simulink model "Paper_2_Model_2_fixed_delay_3_lines"  (R2020b)
settings: Solver=VariableStepAuto  StartTime=0.0  StopTime=3  RelTol=1e-3
libraries: simulink x1
settings Model: Creator=Isabel  LastModifiedBy=Isabel

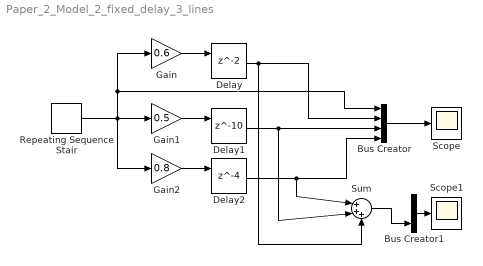
== system Paper_2_Model_2_fixed_delay_3_lines ==
  Bus Creator : BusCreator  Inputs=4
  Bus Creator1 : BusCreator  Inputs=2
  Delay : Delay  InitialConditionSource=Input port  InitialCondition=0  SampleTime=0.01
      settings: InputPortMap=u0,p4
  Delay1 : Delay  DelayLength=10  InitialConditionSource=Input port  InitialCondition=0  SampleTime=0.01
      settings: InputPortMap=u0,p4
  Delay2 : Delay  DelayLength=4  InitialConditionSource=Input port  InitialCondition=0  SampleTime=0.01
      settings: InputPortMap=u0,p4
  Gain : Gain  Gain=0.6
  Gain1 : Gain  Gain=0.5
  Gain2 : Gain  Gain=0.8
  Repeating Sequence Stair : simulink/Sources/Repeating Sequence Stair  OutValues=[0 0 0 1 0 0 0 1 0 0 0 1 0 0 0 1 0 0 0].'  tsamp=0.5  OutMin=[]  OutMax=[]  OutDataTypeStr=double  OutputDataTypeScalingMode=double  OutDataType=fixdt(0,8)  ConRadixGroup=Best Precision: Vector-wise  OutScaling=2^-12
  Scope : Scope
  Scope1 : Scope
  Sum : Sum  Inputs=|+++
  wires:
  Delay/1 -> Sum/3, Bus Creator/2
  Gain1/1 -> Delay1/1
  Gain2/1 -> Delay2/1
  Bus Creator/1 -> Scope/1
  Gain/1 -> Delay/1
  Delay2/1 -> Sum/1, Bus Creator/4
  Repeating Sequence Stair/1 -> Bus Creator/1, Gain/1, Gain2/1, Gain1/1
  Delay1/1 -> Sum/2, Bus Creator/3
  Sum/1 -> Bus Creator1/2
  Bus Creator1/1 -> Scope1/1
